simulink model "Kin_prop_279C_v1"  (R2018b)
settings: Solver=FixedStepAuto  StartTime=0.0  StopTime=1000  FixedStep=.5  RelTol=1e-3
values from neighbouring files (symbols this model uses):
  C = [.892539 .157379 -.422618; -.275451 0.932257 -.234570; .357073 0.325773 .875426]    [PSet3_eml.m]    (also in Pset3_Orbit_prop.m = eye(3); Pset3_Orbit_prop_dim.m = eye(3); gif_test.m)
  DCM = sc.R'*[-1 0 0; 0 -1 0; 0 0 1]    [Compare_run.m]    (also in Pset3_Orbit_prop.m = eye(3); Pset3_Orbit_prop_dim.m = eye(3); Pset_4_TD.m = [0.999999671094767 0 -8.110550887097017e-04; 0 1 0; 8.110550; Sim_Run_File.m)
  I_vec = [sc.Ip(1,1); sc.Ip(2,2); sc.Ip(3,3)]    [Compare_run.m]    (also in PSet2_eml.m; PSet3_eml.m; Pset3_Orbit_prop.m; Pset3_Orbit_prop_dim.m)
  w0 = [1; 1; 1]*pi/180    [Compare_run.m]    (also in Pset3_Orbit_prop.m = [2; 1; 2.5] * pi()/180; Pset3_Orbit_prop_dim.m = [2; 1; 2.5] * pi()/180; Pset_4_TD.m = [omega/100 ; omega;  omega/100]; Sim_Run_File.m = [0.2; 2; 0.2]*pi/180)
settings Model: Creator=Ethan  LastModifiedBy=Ethan

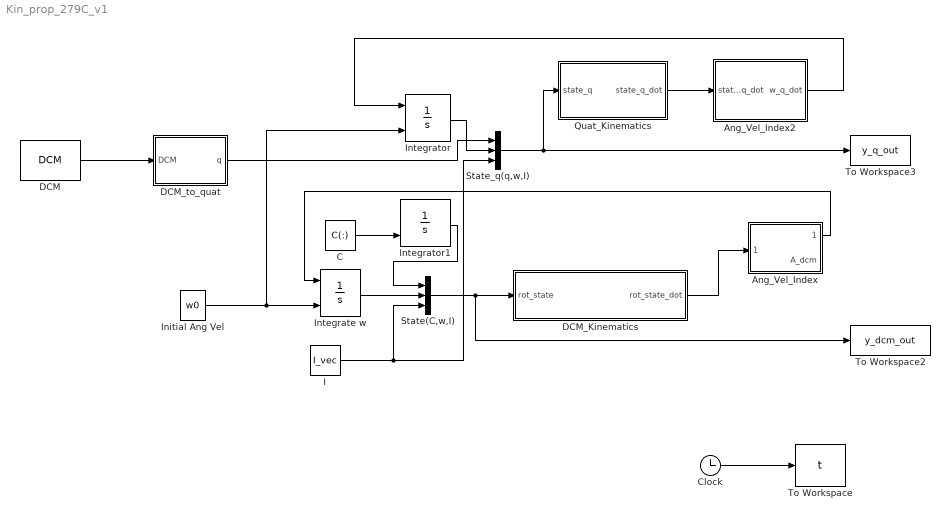
== system Kin_prop_279C_v1 ==
  Ang_Vel_Index : MATLAB Function  TreatAsAtomicUnit=on
  Ang_Vel_Index2 : MATLAB Function  TreatAsAtomicUnit=on
  C : Constant  Value=C(:)
  Clock : Clock
  DCM : Constant  Value=DCM
  DCM_Kinematics : MATLAB Function  TreatAsAtomicUnit=on
  DCM_to_quat : MATLAB Function  TreatAsAtomicUnit=on
  I : Constant  Value=I_vec
  Initial Ang Vel : Constant  Value=w0
  Integrate w : Integrator  InitialConditionSource=external
  Integrator : Integrator  InitialConditionSource=external
  Integrator1 : Integrator  InitialConditionSource=external
  Quat_Kinematics : MATLAB Function  TreatAsAtomicUnit=on
  State(C,w,I) : Concatenate  NumInputs=3
  State_q(q,w,I) : Concatenate  NumInputs=3
  To Workspace : ToWorkspace  VariableName=t  SampleTime=-1
      settings: Save2DSignal=2-D array (concatenate along first dimension)
  To Workspace2 : ToWorkspace  VariableName=y_dcm_out  SampleTime=-1
      settings: Save2DSignal=2-D array (concatenate along first dimension)
  To Workspace3 : ToWorkspace  VariableName=y_q_out  SampleTime=-1
  wires:
  Ang_Vel_Index2/1(w_q_dot) -> Integrator/1
  Quat_Kinematics/1(state_q_dot) -> Ang_Vel_Index2/1(state_q_dot)
  DCM_to_quat/1(q) -> State_q(q,w,I)/1
  Integrator/1 -> State_q(q,w,I)/2
  DCM/1 -> DCM_to_quat/1(DCM)
  DCM_Kinematics/1(rot_state_dot) -> Ang_Vel_Index/1(rot_dcm_dot)
  I/1 -> State(C,w,I)/3, State_q(q,w,I)/3
  State_q(q,w,I)/1 -> Quat_Kinematics/1(state_q), To Workspace3/1
  Ang_Vel_Index/1(w_dcm) -> Integrate w/1
  State(C,w,I)/1 -> To Workspace2/1, DCM_Kinematics/1(rot_state)
  Integrate w/1 -> State(C,w,I)/2
  Initial Ang Vel/1 -> Integrator/2, Integrate w/2
  Clock/1 -> To Workspace/1
  C/1 -> Integrator1/2
  Integrator1/1 -> State(C,w,I)/1

== matlab function Kin_prop_279C_v1/DCM_Kinematics ==
  data: rot_state input; rot_state_dot output
function rot_state_dot  = DCM_kin(rot_state)
% state = [C(:) w1 w2 w3 I1 I2 I3]

rot_state_dot = zeros(length(rot_state),1);
wx = rot_state(10);
wy = rot_state(11);
wz = rot_state(12);
Ix = rot_state(13);
Iy = rot_state(14);
Iz = rot_state(15);
%% Kinematic Equations
Omega = [0 -wz wy; wz 0 -wx; -wy wx 0];
A = [rot_state(1) rot_state(4) rot_state(7); rot_state(2) rot_state(5) rot_state(8); rot_state(3)...
    rot_state(6) rot_state(9)];
rot_state_dot(1:9) = -Omega * A;

%% Euler Equations
rot_state_dot(10) = -wy*wz * (Iz - Iy)/Ix;
rot_state_dot(11) = -wx*wz * (Ix - Iz)/Iy;
rot_state_dot(12) = -wx*wy * (Iy - Ix)/Iz;

end

== matlab function Kin_prop_279C_v1/Ang_Vel_Index ==
  data: rot_dcm_dot input; w_dcm output; A_dcm output
function [w_dcm, A_dcm] = fcn(rot_dcm_dot)

w_dcm = rot_dcm_dot(10:12)';
A_dcm = rot_dcm_dot(1:9)';
end

== matlab function Kin_prop_279C_v1/Quat_Kinematics ==
  data: state_q input; state_q_dot output
function state_q_dot  = quat_kin(state_q)
% state = [q1 q2 q3 q4 w1 w2 w3 I1 I2 I3]

state_q_dot = zeros(length(state_q),1);
wx = state_q(5);
wy = state_q(6);
wz = state_q(7);
%% Kinematic Equations
Omega = [0 wz -wy wx; -wz 0 wx wy; wy -wx 0 wz; -wx -wy -wz 0];
err = 1 - norm(state_q(1:4));
state_q_dot(1:4) = 1/2 * Omega * state_q(1:4) + 0.05 * err * state_q(1:4);

%% Euler Equations
state_q_dot(5) = -wy*wz * (state_q(10) - state_q(9))/state_q(8);
state_q_dot(6) = -wx*wz * (state_q(8) - state_q(10))/state_q(9);
state_q_dot(7) = -wx*wy * (state_q(9) - state_q(8))/state_q(10);

end

== matlab function Kin_prop_279C_v1/DCM_to_quat ==
  data: DCM input; q output
function q  = DCM_to_quat(DCM)
B4 = 1/4 * (1 + trace(DCM));
B1 = 1/4 * (1 + 2*DCM(1,1) - trace(DCM));
B2 = 1/4 * (1 + 2*DCM(2,2) - trace(DCM));
B3 = 1/4 * (1 + 2*DCM(3,3) - trace(DCM));
B = [B1 B2 B3 B4];
[M, I] = max(B);
q = zeros(4,1);
q(4) = sqrt(B(I));
if I == 4
    q(1) = (DCM(2,3) - DCM(3,2)) / 4 / q(4);
    q(2) = (DCM(3,1) - DCM(1,3)) / 4 / q(4);
    q(3) = (DCM(1,2) - DCM(2,1)) / 4 / q(4);
elseif I == 3
    q(2) = (DCM(2,3) + DCM(3,2)) / 4 / q(4);
    q(1) = (DCM(3,1) + DCM(1,3)) / 4 / q(4);
    q(3) = (DCM(1,2) - DCM(2,1)) / 4 / q(4);
elseif I == 2
    q(2) = (DCM(2,3) + DCM(3,2)) / 4 / q(4);
    q(3) = (DCM(3,1) - DCM(1,3)) / 4 / q(4);
    q(1) = (DCM(1,2) + DCM(2,1)) / 4 / q(4);
elseif I == 1
    q(3) = (DCM(2,3) - DCM(3,2)) / 4 / q(4);
    q(2) = (DCM(3,1) + DCM(1,3)) / 4 / q(4);
    q(1) = (DCM(1,2) + DCM(2,1)) / 4 / q(4);
end
q = q/norm(q);
end

== matlab function Kin_prop_279C_v1/Ang_Vel_Index2 ==
  data: state_q_dot input; w_q_dot output
function w_q_dot = fcn(state_q_dot)

w_q_dot = state_q_dot(5:7);

end
